simulink model "zalet_AS"  (R2018b)
settings: Solver=ode4  StartTime=0.0  StopTime=Tsim  FixedStep=Ts  RelTol=1e-3
values from neighbouring files (symbols this model uses):
  J = 0.121970    (= 0.12197)    [skripta_zalet_as.m]
  Vn = 230    [skripta_zalet_as.m]
  Xls = 1.7285    [skripta_zalet_as.m]
libraries: fl_lib x10, nesl_utility x6, pe_lib x4
settings Model: Creator=student  LastModifiedBy=student

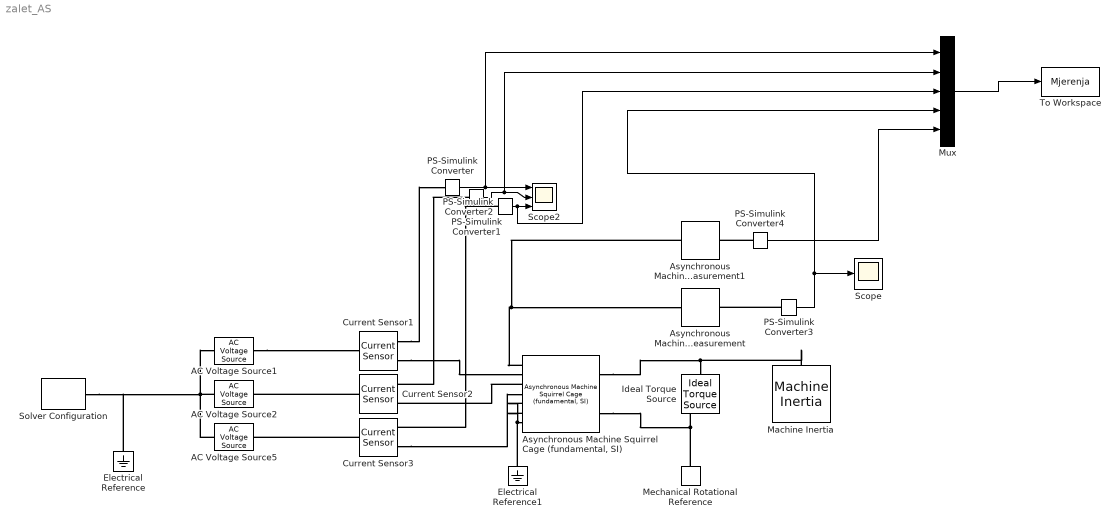
== system zalet_AS ==
  AC Voltage Source1 : fl_lib/Electrical/Electrical Sources/AC Voltage Source  amp=Vn*sqrt(2) V  shift=0 rad  frequency=50 Hz  omega=0 rad/s
  AC Voltage Source2 : fl_lib/Electrical/Electrical Sources/AC Voltage Source  amp=Vn*sqrt(2) V  shift=-2*pi/3 rad  frequency=50 Hz  omega=0 rad/s
  AC Voltage Source5 : fl_lib/Electrical/Electrical Sources/AC Voltage Source  amp=Vn*sqrt(2) V  shift=2*pi/3 rad  frequency=50 Hz  omega=0 rad/s
  Asynchronous Machine Measurement : pe_lib/Machines/Asynchronous Machine Measurement  output_idx=1
      settings: SourceProductName=Simscape Power Systems  SourceProductBaseCode=PS
  Asynchronous Machine Measurement1 : pe_lib/Machines/Asynchronous Machine Measurement  output_idx=2
      settings: SourceProductName=Simscape Power Systems  SourceProductBaseCode=PS
  "Asynchronous Machine Squirrel Cage (fundamental, SI)" : pe_lib/Machines/Asynchronous Machine (Squirrel Cage)/Asynchronous Machine Squirrel Cage (fundamental, SI)  SRated=Sn V*A  VRated=Vn*sqrt(3) V  FRated=f Hz  nPolePairs=p  squirrel_cage=1  zero_sequence=pe.enum.park.zerosequence.exclude  Rs=Rs Ohm  Xls=Xls Ohm  Rrd=Rr Ohm  Xlrd=Xlr Ohm  Rrd1=0.28 Ohm  Xlrd1=0.82 Ohm  Rrd2=0.28 Ohm  Xlrd2=0.82 Ohm  Xm=Xm Ohm  X0=Xls Ohm  saturation_option=0  saturation_i=[0, 4, 9, 18, 25, 34, 50, 68, 95, 120] A  saturation_v=[0, 88, 154, 198, 220, 242, 264, 286, 308, 330] V  connection_option=pe.Connection.delta  param_option=pe.Parameterization.SI  angular_position_specify=off  angular_position_priority=None  angular_position=0 deg  angular_position_nominal_specify=off  angular_position_nominal_unit=deg  angular_position_nominal_value=1  psids_specify=off  psids_priority=None  psids=0 Wb  psids_nominal_specify=off  psids_nominal_unit=Wb  psids_nominal_value=1  psiqs_specify=off  psiqs_priority=None  psiqs=0 Wb  psiqs_nominal_specify=off  psiqs_nominal_unit=Wb  psiqs_nominal_value=1  psi0s_specify=off  psi0s_priority=None  psi0s=0 Wb  psi0s_nominal_specify=off  psi0s_nominal_unit=Wb  psi0s_nominal_value=1
      settings: SourceProductName=Simscape Power Systems  SourceProductBaseCode=PS
  Current Sensor1 : fl_lib/Electrical/Electrical Sensors/Current Sensor
  Current Sensor2 : fl_lib/Electrical/Electrical Sensors/Current Sensor
  Current Sensor3 : fl_lib/Electrical/Electrical Sensors/Current Sensor
  Electrical Reference : fl_lib/Electrical/Electrical Elements/Electrical Reference
  Electrical Reference1 : fl_lib/Electrical/Electrical Elements/Electrical Reference
  Ideal Torque Source : fl_lib/Mechanical/Mechanical Sources/Ideal Torque Source
  Machine Inertia : pe_lib/Machines/Machine Inertia  SRated=Sn V*A  FRated=f Hz  nPolePairs=p  inertia_option=1  J=J kg*m^2  H=3.525 s*W/V/A  damper_option=2  D=39.0509 N*m/(rad/s)  pu_D=0  initialization_option=1  fMechanical0=0 Hz  fElectrical0=0 Hz
      settings: SourceProductName=Simscape Power Systems  SourceProductBaseCode=PS
  Mechanical Rotational Reference : fl_lib/Mechanical/Rotational Elements/Mechanical Rotational Reference
  Mux : Mux  Inputs=5
  PS-Simulink Converter{,1..4} (5 alike) : nesl_utility/PS-Simulink Converter  PhysicalDomain=network_engine_domain  SubClassName=ps_output  LeftPortType=input  RightPortType=output  PseudoPeriodic=off  Frequencies=[]  Unit=1  AffineConversion=off
  Scope : Scope
  Scope2 : Scope  NumInputPorts=3
  Solver Configuration : nesl_utility/Solver Configuration  PhysicalDomain=network_engine_domain  SubClassName=solver  LeftPortType=input  RightPortType=generic  Tones=[]  Harmonics=[]  SimulateNoise=off  Profile=off  UseLocalSampling=off  EnableSwitchedLinearOptims=on  FrequencyDomain=off  UseCCode=off  RelTol=0.001  AbsTol=1e-06  MinStep=1e-09  ToWorkspace=off  RevertToSquareIcSolve=off  NumHomotopyIterations=100  PhasorMode=off  PhasorModeNumHarmonics=1  DoDC=off  ResidualTolerance=1e-09  UseLocalSolver=on  LocalSolverChoice=NE_BACKWARD_EULER_ADVANCER  LocalSolverSampleTime=Ts  DoFixedCost=on  MaxNonlinIter=6  MaxModeIter=2  LinearAlgebra=auto  EquationFormulation=NE_TIME_EF  DelaysMemoryBudget=1024  AutomaticFiltering=on  FilteringTimeConstant=0.001  PartitionStorageMethod=AS_NEEDED  PartitionMemoryBudget=1024
  To Workspace : ToWorkspace  VariableName=Mjerenja  SampleTime=-1
  wires:
  PS-Simulink Converter/1 -> Mux/1, Scope2/1
  PS-Simulink Converter2/1 -> Mux/3, Scope2/3
  PS-Simulink Converter1/1 -> Mux/2, Scope2/2
  PS-Simulink Converter3/1 -> Mux/4, Scope/1
  Mux/1 -> To Workspace/1
  PS-Simulink Converter4/1 -> Mux/5
  connections:
  AC Voltage Source2/RConn1 -- Solver Configuration/RConn1 -- Electrical Reference/LConn1 -- AC Voltage Source5/RConn1 -- AC Voltage Source1/RConn1
  Current Sensor3/LConn1 -- AC Voltage Source5/LConn1
  Current Sensor2/LConn1 -- AC Voltage Source2/LConn1
  AC Voltage Source1/LConn1 -- Current Sensor1/LConn1
  Current Sensor1/RConn2 -- "Asynchronous Machine Squirrel Cage (fundamental, SI)"/RConn2
  "Asynchronous Machine Squirrel Cage (fundamental, SI)"/RConn3 -- Current Sensor2/RConn2
  Current Sensor3/RConn2 -- "Asynchronous Machine Squirrel Cage (fundamental, SI)"/RConn4
  Electrical Reference1/LConn1 -- "Asynchronous Machine Squirrel Cage (fundamental, SI)"/RConn6 -- "Asynchronous Machine Squirrel Cage (fundamental, SI)"/RConn5 -- "Asynchronous Machine Squirrel Cage (fundamental, SI)"/RConn7
  "Asynchronous Machine Squirrel Cage (fundamental, SI)"/LConn1 -- Machine Inertia/LConn1 -- Ideal Torque Source/LConn1
  "Asynchronous Machine Squirrel Cage (fundamental, SI)"/LConn2 -- Mechanical Rotational Reference/LConn1 -- Ideal Torque Source/RConn2
  Current Sensor1/RConn1 -- PS-Simulink Converter/LConn1
  PS-Simulink Converter2/LConn1 -- Current Sensor3/RConn1
  PS-Simulink Converter1/LConn1 -- Current Sensor2/RConn1
  "Asynchronous Machine Squirrel Cage (fundamental, SI)"/RConn1 -- Asynchronous Machine Measurement1/LConn1 -- Asynchronous Machine Measurement/LConn1
  PS-Simulink Converter3/LConn1 -- Asynchronous Machine Measurement/RConn1
  PS-Simulink Converter4/LConn1 -- Asynchronous Machine Measurement1/RConn1
